simulink model "Mo_Hinh_DC_motor_1vong_dk"  (R2019a)
settings: Solver=VariableStepAuto  StartTime=0.0  StopTime=1  RelTol=1e-3
values from neighbouring files (symbols this model uses):
  J = 0.36    [Thong_so_dong_co_1_chieu.m]
  K1oc = 0.1    [Thong_so_dong_co_1_chieu.m]
  Kcp = 10    [Thong_so_dong_co_1_chieu.m]
  Ke = 30*(Ua-Ra*Ia)/(pi*n)    (= 0.339713042931)    [Thong_so_dong_co_1_chieu.m]
  Ki = Kp/T2    [Thong_so_dong_co_1_chieu.m]
  Km = M/Ia    (= 0.255784729969)    [Thong_so_dong_co_1_chieu.m]
  Kp = (T2*Ke)/(2*T1*Kcp*K1oc)    [Thong_so_dong_co_1_chieu.m]
  Ra = 0.585    [Thong_so_dong_co_1_chieu.m]    (also in mTinh_Toan_Thong_so.m = 0.2305)
  Ta = La/Ra    (= 0.0427522435656)    [Thong_so_dong_co_1_chieu.m]
libraries: powerlib x1
settings Model: Creator=Admin  LastModifiedBy=Admin

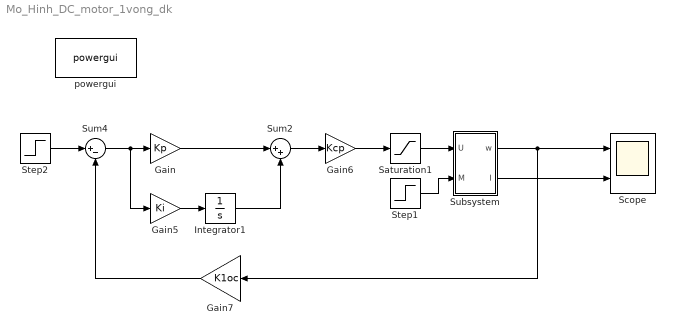
== system Mo_Hinh_DC_motor_1vong_dk ==
  Gain : Gain  Gain=Kp
  Gain5 : Gain  Gain=Ki
  Gain6 : Gain  Gain=Kcp
  Gain7 : Gain  Gain=K1oc
  Integrator1 : Integrator
  Saturation1 : Saturate  UpperLimit=110  LowerLimit=-110
  Scope : Scope  NumInputPorts=2
  Step1 : Step  SampleTime=0
  Step2 : Step  Time=0  After=0.1  SampleTime=0
  Subsystem : Subsystem
  Sum2 : Sum  Inputs=|++
  Sum4 : Sum  Inputs=|+-
  powergui : powerlib/powergui  Priority=1  SimulationMode=Continuous  SampleTime=50e-6  frequency=60  Iterations=50  frequencyindice=60  Pbase=100e6  ErrMax=1e-4  UnitsV=kV  UnitsW=MW  buscounter=0  FunctionMessages=off  echomessages=off  EnableUseOfTLC=off  CurrentSourceSwitches=off  DisableSnubberDevices=off  DisableRonSwitches=off  DisableVfSwitches=off  DisplayEquations=off  AutomaticDiscreteSolvers=off  SolverType=Tustin/Backward Euler (TBE)  Interpol=off  ExternalGateDelay=off  methode=off  Ts=100  x0status=blocks  SPID=on  SwTol=0  HookPort=off  NonlinearTolerance=0  nMaxIteration=15  ContinueOnMaxIteration=off  RestoreLinks=warning  ResistiveCurrentMeasurement=off  Frange=[0:2:500]  Ylog=off  Xlog=on  ShowGrid=off  save=off  variable=ZData  structure=0  ZoomFFT=off  StartTime=0.0  cycles=1  DisplayStyle=1  fundamental=60  FreqAxis=off  MaxFrequency=1000  frequencyindicesteady=1  RmsSteady=1  display=off
      settings: SourceProductName=Simscape Electrical
  wires:
  Gain5/1 -> Integrator1/1
  Gain/1 -> Sum2/1
  Integrator1/1 -> Sum2/2
  Sum2/1 -> Gain6/1
  Gain6/1 -> Saturation1/1
  Sum4/1 -> Gain5/1, Gain/1
  Saturation1/1 -> Subsystem/1(U)
  Step1/1 -> Subsystem/2(M)
  Step2/1 -> Sum4/1
  Subsystem/1(w) -> Gain7/1, Scope/1
  Subsystem/2(I) -> Scope/2
  Gain7/1 -> Sum4/2

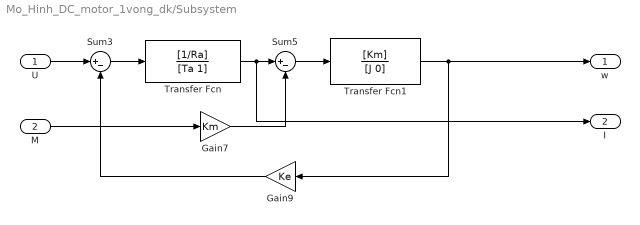
== system Mo_Hinh_DC_motor_1vong_dk/Subsystem ==
  U : Inport
  M : Inport  Port=2
  Gain7 : Gain  Gain=Km
  Gain9 : Gain  Gain=Ke
  Sum3 : Sum  Inputs=|+-
  Sum5 : Sum  Inputs=|+-
  Transfer Fcn : TransferFcn  Numerator=[1/Ra]  Denominator=[Ta 1]
  Transfer Fcn1 : TransferFcn  Numerator=[Km]  Denominator=[J 0]
  w : Outport
  I : Outport  Port=2
  wires:
  Transfer Fcn1/1 -> w/1, Gain9/1
  Sum3/1 -> Transfer Fcn/1
  Sum5/1 -> Transfer Fcn1/1
  Transfer Fcn/1 -> I/1, Sum5/1
  Gain9/1 -> Sum3/2
  Gain7/1 -> Sum5/2
  M/1 -> Gain7/1
  U/1 -> Sum3/1
